simulink model "regcontrol_model_3ph_old"  (R2018b)
settings: Solver=VariableStepAuto  StartTime=0.0  StopTime=10.0  RelTol=1e-3
values from neighbouring files (symbols this model uses):
  BandWidth = Simulink.Parameter    [start.m]
  BaseVoltage = Simulink.Parameter    [start.m]
  CogenEnabled = false    [regcontrol_emulator.m]    (also in start.m = Simulink.Parameter)
  FPTphase = Simulink.Parameter(FPTphases.DEFAULT)    [regcontrol_emulator.m]    (also in start.m = 1)
  IsReversible = Simulink.Parameter    [start.m]
  LDC_Z = Simulink.Parameter    [start.m]
  MaxTap = 1.10    (= 1.1)    [Transformer.m]
  MinTap = 0.90    (= 0.9)    [Transformer.m]
  PTratio = Simulink.Parameter    [start.m]
  R = 0    [start.m]
  RevBand = Simulink.Parameter    [start.m]
  RevVreg = Simulink.Parameter    [start.m]
  TapLimitPerChange = Simulink.Parameter    [start.m]
  UsingRegulatedBus = Simulink.Parameter    [start.m]
  Vlimit = Simulink.Parameter    [start.m]
  Vreg = Simulink.Parameter    [start.m]
  X = 0    [start.m]
undefined symbols (not defined in the file or in its folder): ControlledTransformerConnection, ControlledTransformerCurrents, ControlledTransformerPowers, ControlledTransformerVoltages, ControlModes, CTRating, IsInverseTime, m, n, NumConductors, NumPhases, PresentTap, RevDelay, revLDC_Z, RevPowerThreshold, revR, revX, TapDelay, TapIncrement, TapWinding, TimeDelay, VTerminal
(part 2 of 4)

== stateflow chart regcontrol_model_3ph_old/Queue Handler ==
  settings: enableNonTerminalStates=1
  state Executive [parallel]
    settings: executionOrder=1
    state Asleep
      ex: Status.data = Statuses.READY; % reset status
      INTERNAL_DONE = false;
      EXECUTIVE_DONE = false;
    state DoNearestActions
      state WaitOnPeek
        en: send(QUEUE_PEEK, Internal);
      state WaitOnPop
        en: send(QUEUE_POP, Internal);
      state ErrorNoItems
        en: Status.data = ...
        Statuses.ERROR;
        send(Status);
      (default) -> (junction 302) : % do only those actions with the same delay time as the first action time return time
          | {q_len_initial = GetQueueSize;
          | PendingActionsCompleted = false; % local for now
          | }
      (junction 302) -> (junction 315) [order 1] : [q_len_initial > 0]
      (junction 302) -> Executive.DoNearestActions.ErrorNoItems [order 2]
      (junction 315) -> WaitOnPeek : {INTERNAL_DONE = false;
          | ActionTime = uint8(ExternalAT(DeviceNumber)); % peek with given AT
          | }
      (junction 301) -> (junction 331) [order 1] : [jj <= q_len_initial]
      (junction 331) -> Executive.DoNearestActions.WaitOnPop : {INTERNAL_DONE = false;}
      WaitOnPeek -> (junction 301) : [INTERNAL_DONE]
          | {ActionTime = uint8(Out(QF.Time));
          | QHour = Out(QF.Hour);
          | QSec = Out(QF.Sec);
          | jj = 1;}
      Executive.DoNearestActions.WaitOnPop -> (junction 299) : [INTERNAL_DONE]
          | %send(DoPendingAction);
      (junction 299) -> (junction 301) : {jj = jj + 1;}
      (junction 301) -> (junction 305) [order 2]
      Executive.DoNearestActions.ErrorNoItems -> (junction 300)
      (junction 305) -> (junction 300)
      (junction 300) -> (junction 298) : {EXECUTIVE_DONE = true;}
    state DoAllActions
      state WaitOnPop
        en: send(QUEUE_POP, Internal);
      state ErrorNoItems
        en: Status.data = ...
        Statuses.ERROR;
        send(Status);
      state Finished
      (default) -> (junction 322) : {q_len_initial = GetQueueSize;}
      (junction 322) -> (junction 321) [order 1] : [q_len_initial ~= 0]
      (junction 322) -> Executive.DoAllActions.ErrorNoItems [order 2]
      (junction 321) -> (junction 326) : {ActionTime = uint8(ExternalAT(DeviceNumber));
          | jj = 1;}
      (junction 326) -> (junction 316) [order 1] : [jj <= q_len_initial]
      (junction 316) -> Executive.DoAllActions.WaitOnPop : {INTERNAL_DONE = false;}
      (junction 314) -> (junction 326) : {jj = jj + 1;}
      (junction 326) -> (junction 312) [order 2]
      Executive.DoAllActions.WaitOnPop -> (junction 314) : [INTERNAL_DONE]
          | %send(DoPendingAction);
      Executive.DoAllActions.ErrorNoItems -> (junction 324)
      (junction 312) -> (junction 324)
      (junction 324) -> Finished : {EXECUTIVE_DONE = true;}
    state Pushing1
      en: DeviceNumber = 1;
      send(QUEUE_PUSH, Internal);
    state Pushing2
      en: DeviceNumber = 2;
      send(QUEUE_PUSH, Internal);
    state Pushing3
      en: DeviceNumber = 3;
      send(QUEUE_PUSH, Internal);
    state Pushing
      en: DeviceNumber = 1;
      send(QUEUE_PUSH, Internal);
    state DeletingByHandle
      en: send(QUEUE_DELETE, Internal);
    state Peeking
      en: send(QUEUE_PEEK, Internal);
    state Popping
      en: send(QUEUE_POP, Internal);
    state ReadyAgain
      Status.data = Statuses.READY;
      send(Status);
    (default) -> Executive.Asleep
    Executive.Asleep -> Executive.DeletingByHandle [order 6] : QueueAction[QueueAction.data == ...
        | QueueActions.DELETE]
    Executive.Asleep -> Pushing3 [order 9] : QueueAction[QueueAction.data == ...
        | QueueActions.PUSH_3]
    Executive.Asleep -> Executive.Peeking [order 5] : QueueAction[QueueAction.data == ...
        | QueueActions.PEEK]
    Executive.Asleep -> Pushing2 [order 8] : QueueAction[QueueAction.data == ...
        | QueueActions.PUSH_2]
    Executive.Asleep -> Executive.Popping [order 4] : QueueAction[QueueAction.data == ...
        | QueueActions.POP]
    Executive.Asleep -> Pushing1 [order 7] : QueueAction[QueueAction.data == ...
        | QueueActions.PUSH_1]
    Executive.Asleep -> Executive.Pushing [order 3] : QueueAction[QueueAction.data == ...
        | QueueActions.PUSH]
    Executive.Asleep -> DoAllActions [order 2] : QueueAction[QueueAction.data == ...
        | QueueActions.DO_ALL_ACTIONS]
    ReadyAgain -> Executive.Asleep
    Executive.Asleep -> DoNearestActions [order 1] : QueueAction[QueueAction.data == DO_NEAREST_ACTIONS]
    Pushing2 -> ReadyAgain : [INTERNAL_DONE]
    Pushing1 -> ReadyAgain : [INTERNAL_DONE]
    Pushing3 -> ReadyAgain : [INTERNAL_DONE]
    Executive.Pushing -> ReadyAgain : [INTERNAL_DONE]
    Executive.Popping -> ReadyAgain : [INTERNAL_DONE]
    Executive.DeletingByHandle -> ReadyAgain : [INTERNAL_DONE]
    Executive.Peeking -> ReadyAgain : [INTERNAL_DONE]
    DoAllActions -> ReadyAgain : [EXECUTIVE_DONE]
    DoNearestActions -> ReadyAgain : [EXECUTIVE_DONE]
  state Internal [parallel]
    settings: executionOrder=2
    state Asleep
    state Popping
      (default) -> (junction 163) : % delete from beginning, t<= ActionTime:
          | {q_len = GetQueueSize;
          | ii = 1;
          | }
      (junction 163) -> (junction 169) [order 1] : [ii <= q_len]
      (junction 169) -> (junction 157)
      (junction 157) -> (junction 158) [order 1] : [GetElemTime(ii) <= ActionTime]
      (junction 157) -> (junction 164) [order 2]
      (junction 158) -> (junction 159) : {Out = GetElem(ii);
          | ReduceQueue(ii);
          | DeviceNumber = Out(1,QF.Device);
          | send(DoPendingAction(DeviceNumber));}
          | % break
      (junction 164) -> (junction 163) : {ii = ii + 1;}
      (junction 163) -> (junction 165) [order 2]
      (junction 159) -> (junction 165)
      (junction 165) -> (junction 640)
      (junction 640) -> (junction 641) [order 1] : [QueueEmpty.data == true]
      (junction 640) -> (junction 642) [order 2]
      (junction 641) -> (junction 643) : {send(QueueEmpty);}
      (junction 643) -> (junction 642)
      (junction 642) -> (junction 644) : {INTERNAL_DONE = true;}
    state DeletingByHandle
      (default) -> (junction 664) : % delete from beginning, t<= ActionTime:
          | {q_len = GetQueueSize;
          | ii = 1;
          | }
      (junction 664) -> (junction 671) [order 1] : [ii <= q_len]
      (junction 671) -> (junction 670)
      (junction 670) -> (junction 665) [order 1] : [GetElemHandle(ii) == ...
          | uint8( ExternalHandle(DeviceNumber) )]
      (junction 670) -> (junction 663) [order 2]
      (junction 665) -> (junction 660) : {Out = GetElem(ii);
          | ReduceQueue(ii);}
          | % break
      (junction 663) -> (junction 664) : {ii = ii + 1;}
      (junction 664) -> (junction 668) [order 2]
      (junction 660) -> (junction 668)
      (junction 668) -> (junction 666)
      (junction 666) -> (junction 658) [order 1] : [QueueEmpty.data == true]
      (junction 666) -> (junction 661) [order 2]
      (junction 658) -> (junction 667) : {send(QueueEmpty);}
      (junction 667) -> (junction 661)
      (junction 661) -> (junction 655) : {INTERNAL_DONE = true;}
    state Pushing
      (default) -> (junction 136) : % insert into queue right before item of greater or equal execution time
          | { % transposing to 1x5 and adding 6th field:
          | q_cand = [ (In(DeviceNumber))' double(DeviceNumber) ];
          | q_len = GetQueueSize; %size(queue, 3);
          | ii = 1;
          | }
      (junction 136) -> (junction 134) [order 1] : [ii <= q_len]
      (junction 134) -> (junction 145)
      (junction 145) -> (junction 146) [order 1] : [q_cand(1,QF.Time) <= GetElemTime(ii)]
      (junction 145) -> (junction 137) [order 2]
      (junction 146) -> (junction 148) : {
          | ExpandQueue(ii);}
          | % break
      (junction 137) -> (junction 136) : {ii = ii + 1;}
      (junction 136) -> (junction 138) [order 2] : {ExpandQueue(q_len+1);}
      (junction 148) -> (junction 138)
      (junction 138) -> (junction 151) : %{send(DONE_PUSHING, Executive.Pushing);}
          | {INTERNAL_DONE = true;}
    state Peeking
      (default) -> (junction 181) : % pop without deletion
          | {q_len = GetQueueSize;
          | ii = 1;
          | }
      (junction 181) -> (junction 187) [order 1] : [ii <= q_len]
      (junction 187) -> (junction 175)
      (junction 175) -> (junction 176) [order 1] : [GetElemTime(ii) <= ActionTime]
      (junction 175) -> (junction 182) [order 2]
      (junction 176) -> (junction 177) : {Out = GetElem(ii);}
          | % break
      (junction 182) -> (junction 181) : {ii = ii + 1;}
      (junction 181) -> (junction 183) [order 2]
      (junction 177) -> (junction 183)
      (junction 183) -> (junction 180) : {INTERNAL_DONE = true;}
    (default) -> Internal.Asleep
    Internal.Asleep -> Internal.Pushing [order 1] : QUEUE_PUSH
    Internal.Pushing -> Internal.Asleep : [INTERNAL_DONE]
    Internal.Asleep -> Internal.Popping [order 2] : QUEUE_POP
    Internal.Popping -> Internal.Asleep : [INTERNAL_DONE]
    Internal.Asleep -> Internal.Peeking [order 3] : QUEUE_PEEK
    Internal.Peeking -> Internal.Asleep : [INTERNAL_DONE]
    Internal.Asleep -> Internal.DeletingByHandle [order 4] : QUEUE_DELETE
    Internal.DeletingByHandle -> Internal.Asleep : [INTERNAL_DONE]
  state QF % Queue Fields [group]
  state qs = GetQueueSize [function]
    (default) -> (junction 686) : {[qs, QueueEmpty.data] = mlGetQueueSize;}
  data: Handle local double =1; Time local double =2; Hour local double =3; Sec local double =4; ActionCode local double =5; Device local double =6; qs function_output; depth function_input; h function_output; qs function_output; qe_data function_output; depth function_input; et function_output; elem function_output; depth function_input; depth function_input; depth function_input; DoPendingAction output boolean size=[3 1] =true; QueueAction input Enum: QueueActions; Status output Enum: Statuses; Out output double size=[1 6]; queue output double size=[1 6 50]; q_len local double =0; PendingActionsCompleted local boolean =false; QHour local double; QSec local double; q_cand local double size=[1 5]; In input double size=5; qwriteflag local boolean =false; ii local uint8; jj local uint8; q_len_initial local double; EXECUTIVE_DONE local boolean =false; INTERNAL_DONE local boolean =false;; ExternalAT input double size=[1 3] =100; ActionTime local uint8; QueueEmpty output boolean =false; ExternalHandle input uint8 size=[3 1]; DeviceNumber local uint8 =1
  events: QUEUE_POP local FUNCTION_CALL_EVENT; QUEUE_PUSH local FUNCTION_CALL_EVENT; QUEUE_PEEK local FUNCTION_CALL_EVENT; QUEUE_DELETE local FUNCTION_CALL_EVENT
  function h = GetElemHandle(depth):
    | function h = GetElemHandle(depth)
    |     hh = zeros(1,1);
    |     if ~isempty(queue)
    |         hh = queue(1,QF.Handle,ii);        
    |     end
    |     h = cast(hh, 'uint8'); % for comparison with ExternalHandle
    | end
  function [qs, qe_data] = mlGetQueueSize:
    | function [qs, qe_data] = mlGetQueueSize
    | %     coder.extrinsic('exist');
    | %     eq = zeros(1,1,'double');
    | %     eq = exist('queue');
    | %     if eq == 1 && ~isempty(queue)
    | %         qs = size(queue, 3);
    | %     else % eq ~= 1 || size == 0
    | %         qs = 0;
    | %     end
    |     if ~qwriteflag % can't read intial value of empty queue, so depend on flag
    |         queue = zeros(1,5);
    |         qs = 0;
    |         qe_data = true;
    |         %QueueEmpty.data = true;
    |         qwriteflag = true;
    |     elseif isequal(queue,zeros(1,5)) % case of empty queue (still 1 element)
    |         qs = 0;
    |         qe_data = true;
    |         %QueueEmpty.data = true;
    |     else
    |         qs = size(queue,3);
    |         qe_data = false;
    |         %QueueEmpty.data = false;
    |     end
    | end
  function et = GetElemTime(depth):
    | function et = GetElemTime(depth)
    |     et = zeros(1,1);
    |     if ~isempty(queue)
    |         et = queue(1,QF.Time,ii);
    |     else
    |     end
    | end
  function elem = GetElem(depth):
    | function elem = GetElem(depth)
    |     elem = zeros(1,5);
    |     elem(1,:) = queue(:,:,depth);
    | end
  function ExpandQueue(depth):
    | function ExpandQueue(depth)
    |     rhs = queue(:,:,depth:q_len); % the RHS of the queue
    |     bigger = zeros(1,5,q_len+1);
    |     bigger(:,:,1:(depth-1)) = queue(:,:,1:(depth-1)); % copy LHS
    |     bigger(:,:,depth) = q_cand; % inserting element at end of LHS
    |     %queue(:,:,depth) = q_cand; 
    |     bigger(:,:, (depth+1):(q_len+1)) = rhs; % tack on RHS again
    |     queue = bigger;
    | end
  function ReduceQueue(depth):
    | function ReduceQueue(depth)
    |     rhs = queue(:,:,(depth+1):q_len); % excluding element at depth
    |     smaller = zeros(1,5,q_len-1);
    |     smaller(:,:,1:(depth-1)) = queue(:,:,1:(depth-1)); % lhs, excl. depth
    |     smaller(:,:,depth:(q_len-1)) = rhs; % tack on rhs
    |     queue = smaller;
    | end

== stateflow chart regcontrol_model_3ph_old/RegControl and Execution 1/RegControl ==
  settings: executeAtInitialization=1
  state ControlFlow [parallel]
    settings: executionOrder=1
    state DetermineReversePendingLookingForward
      state CorrectFalseReversePending
        (default) -> (junction 108)
        (junction 108) -> (junction 109) [order 1] : [FwdPower < (-1*RevPowerThreshold)]
        (junction 108) -> (junction 111) [order 2]
        (junction 109) -> (junction 112) : {ReversePending = true;
            | RevHandle = ...
            | Push(ActionCodes.ACTION_REVERSE, ...
            | RevDelay);
            | }
        (junction 112) -> (junction 111)
      state CorrectTrueReversePending
        (default) -> (junction 804)
        (junction 804) -> (junction 123) [order 1] : [FwdPower >= (-1*RevPowerThreshold)]
        (junction 804) -> (junction 809) [order 2]
        (junction 123) -> (junction 806) : % Reset ReversePending:
            | % Delete RevHandle from ControlQueue
            | {DoActions.data = QueueActions.DELETE;
            | send(DoActions);
            | ReversePending = false;
            | RevHandle = 0;}
        (junction 806) -> (junction 809)
      state Finished
        en: GET_VOLTAGE = true;
      (default) -> (junction 106) : {FwdPower = -1*real( ControlledTransformerPower(ElementTerminal) );}
          | % Should we reverse?
      (junction 106) -> ControlFlow.DetermineReversePendingLookingForward.CorrectFalseReversePending [order 1] : [~ReversePending]
      (junction 106) -> (junction 110) [order 2]
      ControlFlow.DetermineReversePendingLookingForward.CorrectFalseReversePending -> (junction 110)
      (junction 110) -> (junction 120)
      (junction 120) -> ControlFlow.DetermineReversePendingLookingForward.CorrectTrueReversePending [order 1] : [ReversePending]
      (junction 120) -> (junction 122) [order 2]
      ControlFlow.DetermineReversePendingLookingForward.CorrectTrueReversePending -> (junction 122)
      (junction 122) -> ControlFlow.DetermineReversePendingLookingForward.Finished
    state DetermineReversePendingLookingReverseOrCogen
      state CorrectFalseReversePending
        (default) -> (junction 130)
        (junction 130) -> (junction 138) [order 1] : [FwdPower > RevPowerThreshold]
        (junction 130) -> (junction 137) [order 2]
        (junction 138) -> (junction 136) : {ReversePending = true;
            | RevHandle = ...
            | Push(ActionCodes.ACTION_REVERSE, ...
            | RevDelay);
            | RevBackHandle = RevHandle;
            | % RevHandle is doing double duty as
            | % RevBackHandle to reduce number of
            | % output ports
            | }
        (junction 136) -> (junction 137)
      state CorrectTrueReversePending
        (default) -> (junction 154)
        (junction 154) -> (junction 799) [order 1] : [FwdPower <= RevPowerThreshold]
        (junction 154) -> (junction 792) [order 2]
        (junction 799) -> (junction 148) : % Reset ReversePending:
            | {RevHandle = RevBackHandle;
            | ReversePending = false;
            | DoActions.data = QueueActions.DELETE;
            | send(DoActions);
            | RevBackHandle = 0;
            | }
        (junction 148) -> (junction 792)
      state Finished
        en: REV_NEUTRAL = true;
      (default) -> (junction 144) : {FwdPower = -1*real( ControlledTransformerPower(ElementTerminal) );}
          | % If reversed, check if power is back in forward direction
      (junction 144) -> ControlFlow.DetermineReversePendingLookingReverseOrCogen.CorrectFalseReversePending [order 1] : [~ReversePending]
      (junction 144) -> (junction 139) [order 2]
      ControlFlow.DetermineReversePendingLookingReverseOrCogen.CorrectFalseReversePending -> (junction 139)
      (junction 139) -> (junction 147)
      (junction 147) -> ControlFlow.DetermineReversePendingLookingReverseOrCogen.CorrectTrueReversePending [order 1] : [ReversePending]
      (junction 147) -> (junction 151) [order 2]
      ControlFlow.DetermineReversePendingLookingReverseOrCogen.CorrectTrueReversePending -> (junction 151)
      (junction 151) -> ControlFlow.DetermineReversePendingLookingReverseOrCogen.Finished
    state ReverseNeutralCase
      state Finished
        en:
        GET_VOLTAGE = true;
      state Exiting
        en: EXIT = true;
      (default) -> (junction 166)
      (junction 166) -> (junction 155) [order 1] : % tap change not specified as needed:
          | [~ArmedOut]
      (junction 166) -> ControlFlow.ReverseNeutralCase.Finished [order 2]
      (junction 155) -> (junction 160) : {UpdatePendingTapChange(0.0);}
      (junction 160) -> (junction 167) [order 1] : [abs(LocalPresentTap - 1.0) < EPSILON]
      (junction 160) -> Exiting [order 2]
      (junction 167) -> (junction 518) : %{Increment = TapIncrement(TapWinding);
          | %PendingTapChange = round( (1.0 - ...
          | %PresentTap(TapWinding)) / Increment ) * Increment;}
          | {UpdatePendingTapChange(...
          | round( (1.0 - double(TapWinding)) / TapIncrement ) * TapIncrement);
          | }
      (junction 518) -> (junction 519) [order 1] : [PendingTapChange ~= 0.0 && ~ArmedOut]
      (junction 519) -> (junction 521) : {% Push ACTION_TAPCHANGE
          | % to ControlQueue with TapDelay:
          | Push(ActionCodes.ACTION_TAPCHANGE, TapDelay);
          | UpdateArmed(true);}
      (junction 518) -> (junction 520) [order 2]
      (junction 521) -> (junction 520)
      (junction 520) -> (junction 164)
      (junction 164) -> Exiting
    state GetVoltage
      state Finished
        en: DETERMINE_VLOCALBUS = true;
      (default) -> (junction 75)
      (junction 75) -> (junction 76) [order 1] : [UsingRegulatedBus]
      (junction 75) -> ControlFlow.GetVoltage.Finished [order 2] : {VBuffer = ControlledTransformerWindingVoltages;
          | %ControlledTransformer.GetWindingVoltages;
          | Vcontrol = GetControlVoltage;}
      (junction 76) -> (junction 78) : {TransformerConnection = ControlledTransformerConnection;
          | %TransformerConnection = ControlledTransformer.Winding(ElementTerminal).Connection;
          | %Vterminal = ComputeVTerminal;
          | }
      (junction 78) -> ControlFlow.GetVoltage.Finished
    state DetermineVlocalbus
      state Finished
        en: GET_VOLTAGEWLDC = true;
      (default) -> (junction 321)
      (junction 321) -> (junction 322) [order 1] : % Voltage limit for bus connected to regulated winding; default = 0.0 (inactive)
          | [VlimitActive]
      (junction 321) -> ControlFlow.DetermineVlocalbus.Finished [order 2] : {Vlocalbus = 0.0;}
      (junction 322) -> (junction 332)
      (junction 332) -> (junction 333) [order 1] : % when controlled transformer is different from LDC PTransformer
          | [UsingRegulatedBus]
      (junction 332) -> (junction 334) [order 2] : % controlled transformer is
          | % the LDC PTransformer
          | {Vlocalbus = abs(Vcontrol);}
      (junction 333) -> (junction 335) : {%ControlledTransformer.GetWindingVoltages(ElementTerminal, VBuffer);
          | Vlocalbus = abs( VBuffer(1) / PTRatio );}
      (junction 335) -> (junction 334)
      (junction 334) -> (junction 324)
      (junction 324) -> ControlFlow.DetermineVlocalbus.Finished
    state GetVoltageWithLDC
      state RX_LDCmode
        (default) -> (junction 365)
        (junction 365) -> (junction 366) [order 1] : [InReverseMode || InCogenMode]
        (junction 365) -> (junction 367) [order 2] : {VLDC = complex(R, X) * complex( real(ILDC), imag(ILDC) );}
        (junction 366) -> (junction 368) : {VLDC = complex(revR, revX) * complex( real(ILDC), imag(ILDC) );}
        (junction 368) -> (junction 367)
      state Z_LDCmode
        (default) -> (junction 387)
        (junction 387) -> (junction 388) [order 1] : [InReverseMode || InCogenMode]
        (junction 387) -> (junction 389) [order 2] : {Vcontrol = abs(Vcontrol) - abs(ILDC) * LDC_Z;}
        (junction 388) -> (junction 390) : {Vcontrol = abs(Vcontrol) - abs(ILDC) * revLDC_Z;}
        (junction 390) -> (junction 389)
      state Finished
        en: GET_TEST_VALUES = true;
      (default) -> (junction 354) : {%%ControlledElement.GetCurrents(CBuffer);
          | %%Convert current to control current by CTRating:
          | ILDC = ControlledTransformerCurrents( NumConductors*ElementTerminal + ControlledPhase - 1) / CTRating;}
      (junction 354) -> RX_LDCmode [order 1] : % Standard R, X LDC
          | [LDC_Z == 0.0]
      (junction 354) -> Z_LDCmode [order 2] : % Beckwith LDC_Z control mode
      Z_LDCmode -> ControlFlow.GetVoltageWithLDC.Finished
      RX_LDCmode -> ControlFlow.GetVoltageWithLDC.Finished
    state GetTestValues
      state Finished
        en:
        DETERMINE_TAP_CHANGE = true;
      (default) -> (junction 398) : % assumes looking forward:
          | {Vactual = abs(Vcontrol);}
      (junction 398) -> (junction 399) [order 1] : [InReverseMode]
      (junction 398) -> ControlFlow.GetTestValues.Finished [order 2] : {VregTest = Vreg;
          | BandTest = Bandwidth;}
      (junction 399) -> (junction 401) : {Vactual = Vactual / LocalPresentTap;
          | VregTest = RevVreg;
          | BandTest = RevBandwidth;}
      (junction 401) -> ControlFlow.GetTestValues.Finished
    state DetermineTapChangeIsNeeded
      state Finished
        en:
        MAKE_TAP_CHANGE = true;
      (default) -> (junction 409)
      (junction 409) -> (junction 410) [order 1] : % difference between desired and actual > half bandwidth
          | [abs(VregTest - Vactual) > BandTest/2.0]
      (junction 409) -> ControlFlow.DetermineTapChangeIsNeeded.Finished [order 2] : {TapChangeIsNeeded = false;}
      (junction 410) -> (junction 412) : {TapChangeIsNeeded = true;}
      (junction 412) -> ControlFlow.DetermineTapChangeIsNeeded.Finished
    state MakeTapChange
      state GetVboostFromVlimit
        (default) -> (junction 441)
        (junction 441) -> (junction 446) [order 1] : [Vlocalbus > Vlimit]
        (junction 441) -> (junction 443) [order 2]
        (junction 446) -> (junction 445) : {Vboost = Vlimit - Vlocalbus;}
        (junction 445) -> (junction 443)
      state TapChangeUp
        (default) -> (junction 475)
        (junction 475) -> (junction 476) [order 1] : [LocalPresentTap < MaxTap]
        (junction 475) -> (junction 477) [order 2]
        (junction 476) -> (junction 478) : {% push ACTION_TAPCHANGE to ControlQueue
            | % with delay ComputeTimeDelay(Vactual):
            | Push(ActionCodes.ACTION_TAPCHANGE, ...
            | ComputeTimeDelay(Vactual));
            | UpdateArmed(true);}
        (junction 478) -> (junction 477)
      state TapChangeDown
        (default) -> (junction 488) : % going down:
        (junction 488) -> (junction 489) [order 1] : [LocalPresentTap > MinTap]
        (junction 488) -> (junction 490) [order 2]
        (junction 489) -> (junction 491) : {% push ACTION_TAPCHANGE to ControlQueue
            | % with delay ComputeTimeDelay(Vactual):
            | Push(ActionCodes.ACTION_TAPCHANGE, ...
            | ComputeTimeDelay(Vactual));
            | UpdateArmed(true);}
        (junction 491) -> (junction 490)
      state Finished
        en: FINISHED = true;
      (default) -> (junction 431) : % compute tapchange:
          | {Vboost = VregTest - Vactual;}
      (junction 431) -> (junction 432) [order 1] : [VlimitActive]
      (junction 431) -> (junction 433) [order 2]
      (junction 432) -> GetVboostFromVlimit
      GetVboostFromVlimit -> (junction 434)
      (junction 434) -> (junction 433)
      (junction 433) -> (junction 435) : {% PU winding boost needed:
          | BoostNeeded = Vboost * PTRatio / BaseVoltage;
          | Increment = TapIncrement(TapWinding);
          | % quantize to an increment:
          | UpdatePendingTapChange( ...
          | round(BoostNeeded/Increment)*Increment);
          | }
      (junction 435) -> (junction 453) : % send initial tap change message to ControlQueue, add delay time to solution control queue:
      (junction 453) -> (junction 454) [order 1] : % only changes 1 tap at a time:
          | [PendingTapChange ~= 0.0 && ~ArmedOut]
      (junction 453) -> ControlFlow.MakeTapChange.Finished [order 2]
      (junction 454) -> (junction 464) : % see of any tap change is possible in desired direction (not saturated):
      (junction 464) -> TapChangeUp [order 1] : % going up:
          | [PendingTapChange > 0.0]
      (junction 464) -> TapChangeDown [order 2]
      TapChangeUp -> (junction 467)
      TapChangeDown -> (junction 466)
      (junction 467) -> (junction 466)
      (junction 466) -> (junction 456)
      (junction 456) -> ControlFlow.MakeTapChange.Finished
    state Finished
    (default) -> (junction 207) : {AssignInputsToLocals();
        | ResetTransitionFlags();}
    (junction 207) -> (junction 208) [order 2]
    (junction 208) -> (junction 86)
    (junction 207) -> (junction 529) [order 1] : [TapLimitPerChange == 0]
    (junction 86) -> (junction 87) [order 1] : [~UsingRegulatedBus]
    (junction 87) -> (junction 61)
    (junction 86) -> (junction 88) [order 2]
    (junction 61) -> (junction 62) [order 1] : [IsReversible || CogenEnabled]
    (junction 61) -> (junction 65) [order 2]
    (junction 62) -> (junction 63)
    (junction 63) -> DetermineReversePendingLookingForward [order 1] : [LookingForward && ~InCogenMode]
    (junction 63) -> DetermineReversePendingLookingReverseOrCogen [order 2]
    DetermineReversePendingLookingForward -> (junction 67) : [GET_VOLTAGE]
    DetermineReversePendingLookingReverseOrCogen -> (junction 175) : [REV_NEUTRAL]
    (junction 175) -> ReverseNeutralCase [order 1] : % mode for which tap change may be executed,
        | % but no reversal made:
        | [ReverseNeutral]
    (junction 175) -> (junction 174) [order 2]
    ReverseNeutralCase -> (junction 174) [order 2] : [GET_VOLTAGE]
    (junction 174) -> (junction 127)
    ReverseNeutralCase -> (junction 532) [order 1] : [EXIT]
    (junction 65) -> (junction 88)
    (junction 127) -> (junction 65)
    (junction 67) -> (junction 127)
    (junction 88) -> GetVoltage
    (junction 532) -> (junction 529)
    (junction 529) -> (junction 212)
    GetVoltage -> DetermineVlocalbus : [DETERMINE_VLOCALBUS]
    DetermineVlocalbus -> (junction 343) : [GET_VOLTAGEWLDC]
    (junction 343) -> GetVoltageWithLDC [order 1] : % line drop compensation, but not using regulated bus
        | [~UsingRegulatedBus && LDCActive]
    (junction 343) -> (junction 345) [order 2]
    GetVoltageWithLDC -> (junction 346) : [GET_TEST_VALUES]
    (junction 346) -> (junction 345)
    (junction 345) -> GetTestValues
    GetTestValues -> DetermineTapChangeIsNeeded : [DETERMINE_TAP_CHANGE]
    DetermineTapChangeIsNeeded -> (junction 420) : [MAKE_TAP_CHANGE]
    (junction 420) -> MakeTapChange [order 1] : [TapChangeIsNeeded]
    (junction 420) -> (junction 422) [order 2]
    MakeTapChange -> (junction 423) : [FINISHED]
    (junction 423) -> (junction 422)
    (junction 422) -> ControlFlow.Finished
    (junction 212) -> ControlFlow.Finished : {UpdatePendingTapChange(0);}
  state UpdateLocals [parallel]
    settings: executionOrder=2
    state Asleep
      ex: UPDATED = false;
    state UpdatePresentTap
      en: LocalPresentTap = ...
      PresentTap;
      ex: UPDATED = true;
    state UpdateArmed
      en: ArmedOut = ArmedIn;
      ex: UPDATED = true;
    state UpdateHandle
      en:
      if HandleIn > HandleOut
      HandleOut = HandleIn;
      end
      ex: UPDATED = true;
    (default) -> Asleep
    Asleep -> UpdateHandle [order 3] : UpdateRegControl[UpdateRegControl.data == ...
        | UpdateActions.HANDLE]
    Asleep -> UpdatePresentTap [order 1] : UpdateRegControl[UpdateRegControl.data == ...
        | UpdateActions.PRESENT_TAP]
    UpdatePresentTap -> Asleep : [UPDATED]
    UpdateHandle -> Asleep : [UPDATED]
    Asleep -> UpdateArmed [order 2] : UpdateRegControl[UpdateRegControl.data == ...
        | UpdateActions.ARMED]
    UpdateArmed -> Asleep : [UPDATED]
  state UpdatePendingTapChange(Change) [function]
    (default) -> (junction 1030) : {
        | PendingTapChange = Change;
        | UpdateExecution.data = ...
        | UpdateActions.PENDING_TAPCHANGE;
        | send(UpdateExecution);
        | }
  state UpdateArmed(NewArmed) [function]
    (default) -> (junction 1031) : {
        | ArmedOut = NewArmed;
        | UpdateExecution.data = ...
        | UpdateActions.ARMED;
        | send(UpdateExecution);
        | }
  state AssignInputsToLocals [function]
    (default) -> (junction 987) : {BandWidth = Equipment.BandWidth;
        | UsingRegulatedBus = Equipment.UsingRegulatedBus;
        | CogenEnabled = Equipment.CogenEnabled;
        | LDC_Z = Equipment.LDC_Z;
        | TapLimitPerChange = Equipment.TapLimitPerChange;
        | PTratio = Equipment.PTratio;
        | RevBand = Equipment.RevBand;
        | RevDelay = Equipment.RevDelay;
        | IsReversible = Equipment.IsReversible;
        | RevVreg = Equipment.RevVreg;
        | RevPowerThreshold = Equipment.RevPowerThreshold;
        | Vlimit = Equipment.Vlimit;
        | Vreg = Equipment.Vreg;
        | TapDelay = Equipment.TapDelay;
        | TapWinding = Equipment.TapWinding;
        | FPTphase = Equipment.FPTphase;
        |
        | MinTap = Equipment.MinTap;
        | MaxTap = Equipment.MaxTap;
        | TapIncrement = Equipment.TapIncrement;
        | ControlledTransformerConnection = Equipment.ControlledTransformerConnection;
        | BaseVoltage = Equipment.BaseVoltage;
        | NumConductors = Equipment.NumConductors;
        | NumPhases = Equipment.NumPhases;
        | CTRating = Equipment.CTRating;
        | IsInverseTime = Equipment.IsInverseTime;
        |
        | R = Equipment.R;
        | X = Equipment.X;
        | revR = Equipment.revR;
        | revX = Equipment.revX;
        | revLDC_Z = Equipment.revLDC_Z;
        | TimeDelay = Equipment.TimeDelay;
        |
        | % PresentTap = Equipment.PresentTap;
        | % PresentTap's workspace value is evaluated in Execution,
        | % meaning that PresentTap (an input here) is fine without assignment
        |
        | ControlledTransformerWindingVoltages = Signals.ControlledTransformerVoltages;
        | ControlledTransformerPower = Signals.ControlledTransformerPowers;
        | ControlledTransformerCurrents = Signals.ControlledTransformerCurrents;
        | VTerminal = Signals.VTerminal;
        |
        | VBuffer = zeros([length(ControlledTransformerWindingVoltages) 1]);
        | % ArmedOut = ArmedIn;
        | }
    (junction 987) -> (junction 996) [order 1] : [R~=0 || X~=0 || LDC_Z ~=0]
    (junction 987) -> (junction 991) [order 2] : {LDCActive = false;}
    (junction 996) -> (junction 990) : {LDCActive = true;}
    (junction 990) -> (junction 991)
    (junction 991) -> (junction 900)
  state h = Push(CodeVal, DelayVal) [function]
    (default) -> (junction 860) : {ControlAction = CodeVal;
        | Delay = DelayVal;
        | HandleOut = HandleOut + double(1);
        | UpdateRegControl.data = ...
        | UpdateActions.HANDLE;
        | send(UpdateExecution);
        | DoActions.data = QueueActions.PUSH;
        | send(DoActions);
        | h = uint8(HandleOut);}
  note: BandWidth
      | UsingRegulatedBus
      | CogenEnabled
      | LDC_Z
      | TapLimitPerChange
      | PTratio
      | RevBand
      | IsReversible
      | RevVreg
      | Vlimit
      | Vreg
      | ILDC
      | FwdPower
  state ResetTransitionFlags [function]
    (default) -> (junction 886) : {DETERMINE_TAP_CHANGE = false;
        | DETERMINE_VLOCALBUS = false;
        | EXIT = false;
        | FINISHED = false;
        | GET_TEST_VALUES = false;
        | GET_VOLTAGE = false;
        | GET_VOLTAGEWLDC = false;
        | MAKE_TAP_CHANGE = false;
        | REV_NEUTRAL = false;}
  state UpdateControlledTransformerWV [function] [commented out]
    note: Retrieves new value for ControlledTransformerWindingVoltages. Update since last call of AssignInputsToLocals. Necessary because the control flow requires multiple updates to this quantity.
    (default) -> (junction 905) [commented out] : {ControlledTransformerWindingVoltages = ...
        | Inputs.ControlledTransformerWindingVoltages;}
  state UpdateControlledTransformerPower [function] [commented out]
    note: Retrieves new value for ControlledTransformerPower. Update since last call of AssignInputsToLocals. Necessary because the control flow requires multiple updates to this quantity.
    (default) -> (junction 902) [commented out] : {ControlledTransformerPower = ...
        | Inputs.ControlledTransformerPower;}
  state vt = ComputeVTerminal [function] [commented out]
    (default) -> (junction 309) [commented out] : % Iteration through order of admittance matrix
        | % (inherited from CktElement)
    (junction 310) -> (junction 308) [commented out] : [ii <= Yorder]
    (junction 308) -> (junction 311) [commented out] : {vt(ii) = NodeV(NodeRef(ii));}
    (junction 309) -> (junction 310) [commented out] : {ii = 1;}
    (junction 311) -> (junction 310) [commented out] : {ii = ii + 1;}
    (junction 310) -> (junction 312) [commented out]
  state WindingVoltages = GetWindingVoltages(Transformer, IndicatedWinding) [function] [commented out]
    note: Intend to store WindingVoltages in VBuffer.
        | Fills array with voltages across indicated winding
    note: For Delta connections or Line-Line voltages
    (default) -> (junction 969) [commented out] : % Determine whether winding exists
    (junction 923) -> (junction 921) [commented out] : [ii <= Yorder]
    (junction 921) -> (junction 924) [commented out] : {Vterminal(ii) = NodeV( NodeRef(i) );}
    (junction 969) -> (junction 922) [commented out] : [IndicatedWinding >= 1 && IndicatedWinding <= NumWindings]
    (junction 969) -> (junction 971) [commented out]
    (junction 922) -> (junction 923) [commented out] : {ii = 1;}
    (junction 924) -> (junction 923) [commented out] : {ii = ii + 1;}
    (junction 923) -> (junction 925) [commented out] : {k = (IndicatedWinding - 1) * Fnconds;
        | NeutTerm = Fnphases + k + 1;}
    (junction 925) -> (junction 935) [commented out] : {ii = 1;}
    (junction 935) -> (junction 933) [commented out] : [ii <= Fnphases]
    (junction 933) -> (junction 952) [commented out]
    (junction 952) -> (junction 953) [commented out] : [Winding(IndicatedWinding).Connection == Connections.WYE]
    (junction 952) -> (junction 956) [commented out]
    (junction 953) -> (junction 954) [commented out] : {VBuffer(ii) = Vterminal(ii + k) - Vterminal(NeutTerm);}
    (junction 954) -> (junction 955) [commented out]
    (junction 955) -> (junction 959) [commented out]
    (junction 956) -> (junction 957) [commented out] : [Winding(IndicatedWinding).Connection == Connections.DELTA]
    (junction 956) -> (junction 960) [commented out]
    (junction 957) -> (junction 958) [commented out] : {iii = RotatePhases(ii);
        | VBuffer(ii) = ...
        | Vterminal(ii + k) - ...
        | Vterminal(iii+k);}
    (junction 936) -> (junction 935) [commented out] : {ii = ii + 1;}
    (junction 935) -> (junction 937) [commented out] : {WindingVoltages = VBuffer;}
    (junction 958) -> (junction 959) [commented out]
    (junction 959) -> (junction 961) [commented out]
    (junction 961) -> (junction 960) [commented out]
    (junction 960) -> (junction 936) [commented out]
    (junction 937) -> (junction 971) [commented out]
    (junction 971) -> (junction 973) [commented out]
  state Result = GetControlVoltage [function]
    (default) -> (junction 236)
    (junction 236) -> (junction 237) [order 1] : [FPTphase == NumPhases] %MAXPHASE
        | % controlled phase is that with greatest |V|
    (junction 236) -> (junction 240) [order 2]
    (junction 237) -> (junction 260) : {ControlledPhase = 1;
        | % abs is equivalent to Cabs:
        | V = abs( VBuffer(ControlledPhase) );}
        | % Iteration through remaining phases:
    (junction 261) -> (junction 259) [order 1] : [ii <= NumPhases]
    (junction 259) -> (junction 270)
    (junction 260) -> (junction 261) : {ii = uint8(2);}
    (junction 270) -> (junction 271) [order 1] : [abs( VBuffer(ControlledPhase)) > V]
        | % if it's GREATER, make it the new V
    (junction 270) -> (junction 272) [order 2]
    (junction 271) -> (junction 273) : {V = abs( VBuffer(ii) );
        | ControlledPhase = ii;}
    (junction 262) -> (junction 261) : {ii = ii+1;}
    (junction 261) -> (junction 238) [order 2] : {Result = VBuffer(ControlledPhase) / PTRatio;
        | % Complex divided by real
        | }
    (junction 273) -> (junction 272)
    (junction 272) -> (junction 262)
    (junction 238) -> (junction 239)
    (junction 239) -> (junction 243)
    (junction 240) -> (junction 241) [order 1] : [FPTphase == 1] % MINPHASE
        | % controlled phase is that with least |V|
    (junction 240) -> (junction 244) [order 2] : % just use one phase because
        | % that's what most controls do:
        | {Result = VBuffer(FPTphase) / PTRatio;
        | ControlledPhase = FPTphase;}
    (junction 241) -> (junction 282) : {ControlledPhase = 1;
        | % abs is equivalent to Cabs:
        | V = abs( VBuffer(ControlledPhase) );}
        | % Iteration through remaining phases:
    (junction 278) -> (junction 277) [order 1] : [ii <= NumPhases]
    (junction 277) -> (junction 291)
    (junction 282) -> (junction 278) : {ii = uint8(2);}
    (junction 291) -> (junction 292) [order 1] : [abs( VBuffer(ControlledPhase)) < V]
        | % if it's LESS, make it the new V
    (junction 291) -> (junction 293) [order 2]
    (junction 292) -> (junction 294) : {V = abs( VBuffer(ii) );
        | ControlledPhase = ii;}
    (junction 280) -> (junction 278) : {ii = ii+1;}
    (junction 278) -> (junction 242) [order 2] : {Result = VBuffer(ControlledPhase) / PTRatio;
        | % Complex divided by real
        | }
    (junction 294) -> (junction 293)
    (junction 293) -> (junction 280)
    (junction 242) -> (junction 243)
    (junction 243) -> (junction 245)
    (junction 245) -> (junction 244)
    (junction 244) -> (junction 246)
  state Result = ComputeTimeDelay(Vavg) [function]
    (default) -> (junction 507)
    (junction 507) -> (junction 508) [order 1] : [IsInverseTime]
    (junction 507) -> (junction 509) [order 2] : % determines which regulator control will act first,
        | % default is 15s
        | {Result = TimeDelay;}
    (junction 508) -> (junction 510) : % TimeDelay is adjusted inversely proportional to
        | % the amount that voltage is outside the band,
        | % down to 10 percent of specified time delay
        | % (Further out of band = band - 1> less time delay)
        | {Result = TimeDelay / min(10.0, 2.0*abs(Vreg - Vavg)/Bandwidth);}
    (junction 510) -> (junction 509)
    (junction 509) -> (junction 511)
  data: Change function_input; NewArmed function_input; CodeVal function_input; DelayVal function_input; h function_output; vt function_output; IndicatedPhase function_input; RotatedPhase function_output; Transformer function_input; IndicatedWinding function_input; WindingVoltages function_output; Result function_output; Vavg function_input; Result function_output; Signals input Bus: SignalBus; Equipment input Bus: EquipmentBus; BandTest local double =0; BoostNeeded local double =0; Increment local double =0; ReversePending local boolean =false; TapChangeIsNeeded local boolean =false; Vactual local double =0; Vboost local double =0; Vcontrol local double =complex(0); Vlocalbus local double =0; VregTest local double =0; EPSILON local double =1.0e-12; R local double =0; X local double =0; BaseVoltage local double; ControlledPhase local uint8 size=[1]; ElementTerminal local uint8 size=[1] =uint8(1); InCogenMode local boolean =false; InReverseMode local boolean =false; LDCActive local boolean =false; LookingForward local boolean =false; MaxTap local double; MinTap local double; RevPowerThreshold local double; ReverseNeutral local boolean =false; TapIncrement local double; TapWinding local uint8 size=[1] =uint8(1); VBuffer local double size=[4 1]; VlimitActive local boolean =false; revLDC_Z local double =0; revR local double =0; revX local double =0; TransformerConnection local uint8 size=[1] =uint8(0); Bandwidth local double =3; CogenEnabled local boolean =false; FwdPower local double =0; ILDC local double =complex(0); IsReversible local boolean =false; LDC_Z local double =0; PTRatio local double =60; RevBandwidth local double =3; RevVreg local double =120; TapLimitPerChange local uint8 size=[1] =uint8(16); UsingRegulatedBus local boolean =false; Vlimit local double =0; Vreg local double =120; ControlAction output Enum: ActionCodes; ArmedIn input boolean =false; Delay output double =0; HandleOut output =double(0); DoActions output Enum: QueueActions; RevBackHandle local uint8 size=[1] =uint8(0); REV_NEUTRAL local boolean =false; RevDelay local double; ControlledTransformerWindingVoltages local double size=[4 1]; ControlledTransformerConnection local uint8 size=[1]; EXIT local boolean =false; FINISHED local boolean =false; GET_TEST_VALUES local boolean =false; MAKE_TAP_CHANGE local boolean =false; DETERMINE_TAP_CHANGE local boolean =false; GET_VOLTAGE local boolean =false; GET_VOLTAGEWLDC local boolean =false; DETERMINE_VLOCALBUS local boolean =false; TapDelay local double; HandleIn input double; ControlledTransformerPower local double; VLDC local double =complex(0); ControlledTransformerCurrents local double; CTRating local double; NumConductors local uint8 size=[1]; NumPhases local uint8 size=[1]; IsInverseTime local boolean; FPTphase local uint8 size=[1]; TimeDelay local double; RevHandle output uint8 size=[1] =uint8(0); PendingTapChange output double size=[1] =double(0); ArmedOut output boolean =false; LocalPresentTap local double =double(1); PresentTap input double; UpdateRegControl input Enum: UpdateActions; UPDATED local boolean =false; UpdateExecution output Enum: UpdateActions
  function RotatedPhase = RotatePhases(IndicatedPhase):
    | function RotatedPhase = RotatePhases(IndicatedPhase)
    |     HVLeadsLV = false;
    |     % FIRST NEED TO DETERMINE DELTADIRECTION:
    |     % If high voltage is delta, delta leads y (1)
    |     % If high voltage is wye, delta lags wye (2)
    |     if Winding(1).connection == Winding(2).connection
    |         DeltaDirection = 1;
    |     else
    |         if Winding(1).kvll >= Winding(2).kvll
    |             iHvolt = 1;
    |         else
    |             iHVolt = 2;
    |         end
    |         switch Winding(iHvolt).Connection
    |             case 0
    |                 if HVLeadsLV
    |                     DeltaDirection = -1;
    |                 else
    |                     DeltaDirection = 1;
    |                 end
    |             case 1
    |                 if HVLeadsLV
    |                     DeltaDirection = 1;
    |                 else
    |                     DeltaDirection = -1;
    |                 end
    |         end
    |     end
    |     
    |     % NOW, ACTUALLY DETERMINE PHASE ROTATION
    |     RotatedPhase = IndicatedPhase + DeltaDirection;
    | 
    |     % make sure RotatedPhase is within limits:
    |     if fNphases > 2
    |         % Assumes 2 phase delta is open delta
    |         if RotatedPhase > fNphases
    |             RotatedPhase = 1;
    |         elseif RotatedPhase < 1
    |             RotatedPhase = fNphases;
    |         end
    |     elseif RotatedPhase < 1
    |         RotatedPhase = 3; % For 2-phase delta, next phase will be 3rd phase
    |     end
    | end
